simulink model "simAntiWindup"  (R2022b)
settings: Solver=ode15s  StartTime=0.0  StopTime=4*500-1  RelTol=1e-6  EnableMultiTasking=on
libraries: simulink_need_slupdate x2, simulink x2
settings Model: Creator=Adolfo  LastModifiedBy=adolfo
settings SolverCC: MaxConsecutiveZCs=10000  ZeroCrossAlgorithm=Adaptive  AlgebraicLoopSolver=TrustRegion
settings DataIOCC: LimitDataPoints=on  SaveFormat=Array  SignalLoggingSaveFormat=ModelDataLogs  ReturnWorkspaceOutputs=off
settings OptimizationCC: ExpressionDepthLimit=2147483647  InitFltsAndDblsToZero=on  LifeSpan=inf
settings DebuggingCC: SaveWithParameterizedLinksMsg=none  UnderspecifiedInitializationDetection=Classic  MergeDetectMultiDrivingBlocksExec=none  SignalResolutionControl=TryResolveAllWithWarning  SolverPrmCheckMsg=warning  MultiTaskDSMMsg=warning  MultiTaskCondExecSysMsg=none  FcnCallInpInsideContextMsg=warning  UnconnectedInputMsg=warning  UnconnectedOutputMsg=warning  UnconnectedLineMsg=warning  StateNameClashWarn=warning  SFUnexpectedBacktrackingDiag=warning  SFNoUnconditionalDefaultTransitionDiag=warning  SFExecutionAtInitializationDiag=none  SFMachineParentedDataDiag=warning  ArithmeticOperatorsInVariantConditions=warning
settings HardwareCC: ProdBitPerPointer=32  ProdBitPerSizeT=32  ProdBitPerPtrDiffT=32  ProdLargestAtomicFloat=None  ProdIntDivRoundTo=Undefined  ProdEndianess=Unspecified  ProdWordSize=32  ProdHWDeviceType=32-bit Generic
settings ModelReferenceCC: EnableRefExpFcnMdlSchedulingChecks=on  PropagateSignalLabelsOutOfModel=off
settings SFSimCC: SimUseLocalCustomCode=off  CustomCodeUndefinedFunction=UseInterfaceOnly
settings RTWCC: RTWUseLocalCustomCode=off
settings CodeAppCC: StateflowObjectComments=on
settings GRTTargetCC: TargetFcnLib=ansi_tfl_tmw.mat  TargetLangStandard=C89/C90 (ANSI)  CombineOutputUpdateFcns=off  GRTInterface=on
settings ConfigComp: CovMetricSettings=dw  CovSaveCumulativeToWorkspaceVar=on  CovSaveSingleToWorkspaceVar=on  CovExternalEMLEnable=off

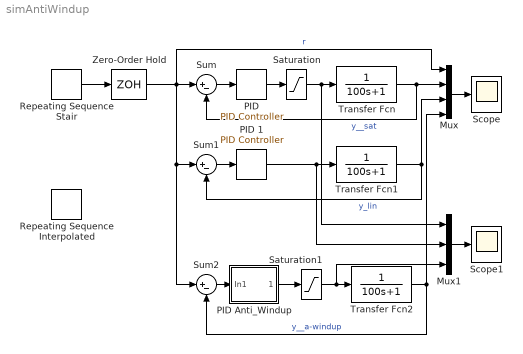
== system simAntiWindup ==
  Mux : Mux
  Mux1 : Mux  Inputs=3
  PID : simulink_need_slupdate/PID Controller  P=10  I=.5  D=10
  PID Anti_Windup : Subsystem
  PID 1 : simulink_need_slupdate/PID Controller  P=10  I=.5  D=10
  Repeating Sequence Interpolated : simulink/Sources/Repeating Sequence Interpolated  OutValues=[0 0 10 10 20 20 30 30 40 40].'  TimeValues=[0 0.1 500 500.1 1000 1000.1 1500 1500.1 2000 2000.1].'  LookUpMeth=Interpolation-Use End Values  tsamp=0.01  OutMin=[]  OutMax=[]  OutDataTypeStr=double  OutputDataTypeScalingMode=double  OutDataType=fixdt(0,8)  OutScaling=2^-10
  Repeating Sequence Stair : simulink/Sources/Repeating Sequence Stair  OutValues=10*[1 2 3 4 5 6].'  tsamp=500  OutMin=[]  OutMax=[]  OutDataTypeStr=float('double')  OutputDataTypeScalingMode=Specify via dialog  OutDataType=float('double')  ConRadixGroup=Best Precision: Vector-wise  OutScaling=2^-12
  Saturation : Saturate  UpperLimit=50  LowerLimit=0
  Saturation1 : Saturate  UpperLimit=50  LowerLimit=0
  Scope : Scope
  Scope1 : Scope
  Sum : Sum  Inputs=|+-
  Sum1 : Sum  Inputs=|+-
  Sum2 : Sum  Inputs=|+-
  Transfer Fcn : TransferFcn  Denominator=[100 1]
  Transfer Fcn1 : TransferFcn  Denominator=[100 1]
  Transfer Fcn2 : TransferFcn  Denominator=[100 1]
  Zero-Order Hold : ZeroOrderHold  SampleTime=-1
  wires:
  Zero-Order Hold/1 -> Sum/1, Sum1/1, Sum2/1, Mux/1  "r"
  Transfer Fcn/1 -> Sum/2, Mux/2  "y__sat"
  PID/1 -> Saturation/1
  Sum/1 -> PID/1
  Saturation/1 -> Transfer Fcn/1, Mux1/1
  Mux/1 -> Scope/1
  Transfer Fcn1/1 -> Sum1/2, Mux/3  "y_lin"
  PID 1/1 -> Transfer Fcn1/1, Mux1/2
  Sum1/1 -> PID 1/1
  Transfer Fcn2/1 -> Sum2/2, Mux/4  "y__a-windup"
  PID Anti_Windup/1(Out1) -> Saturation1/1
  Sum2/1 -> PID Anti_Windup/1(In1)
  Saturation1/1 -> Transfer Fcn2/1, Mux1/3
  Mux1/1 -> Scope1/1
  Repeating Sequence Stair/1 -> Zero-Order Hold/1

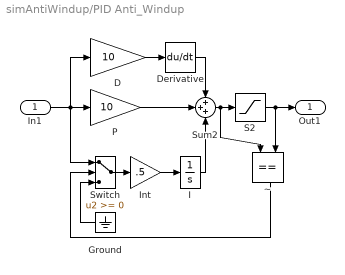
== system simAntiWindup/PID Anti_Windup ==
  In1 : Inport
  D : Gain  Gain=10
  Derivative : Derivative
  Ground : Ground
  I : Integrator
  Int : Gain  Gain=.5
  P : Gain  Gain=10
  S2 : Saturate  UpperLimit=50  LowerLimit=0
  Sum2 : Sum  Inputs=+++
  Switch : Switch  SaturateOnIntegerOverflow=off  InputSameDT=off
  ~ : RelationalOperator  Operator===  OutDataTypeStr=boolean  InputSameDT=off
  Out1 : Outport
  wires:
  S2/1 -> ~/2, Out1/1
  In1/1 -> Switch/1, D/1, P/1
  D/1 -> Derivative/1
  Derivative/1 -> Sum2/1
  P/1 -> Sum2/2
  Switch/1 -> Int/1
  Ground/1 -> Switch/3
  I/1 -> Sum2/3
  Sum2/1 -> S2/1, ~/1
  ~/1 -> Switch/2
  Int/1 -> I/1
